simulink library "cfr_3fir_lib"  (Simulink 8.7)
settings: Solver=ode45  StartTime=0.0  StopTime=10.0  RelTol=1e-3
undefined symbols (not defined in the file): AdvDSPBChannelOutDisplay, Anti, cfr0_id, cfr_Params, clock_rate, dpoly, dspba_ChannelInVis, dspba_ChannelOutVis, dspba_internal_get_channel_ports, evalAionMaskParam, Folding, latency, primtype, REG, REG_dut_id_addr, sample_rate, Symmetrical, value
libraries: DSPBAPrim x83, CORDIC_lib x17, Pipereg_lib x15, DSPBAModelBus x3, DSPBAFilters x3
(part 1 of 2)
settings Model: Creator=nsafari  LastModifiedBy=5g

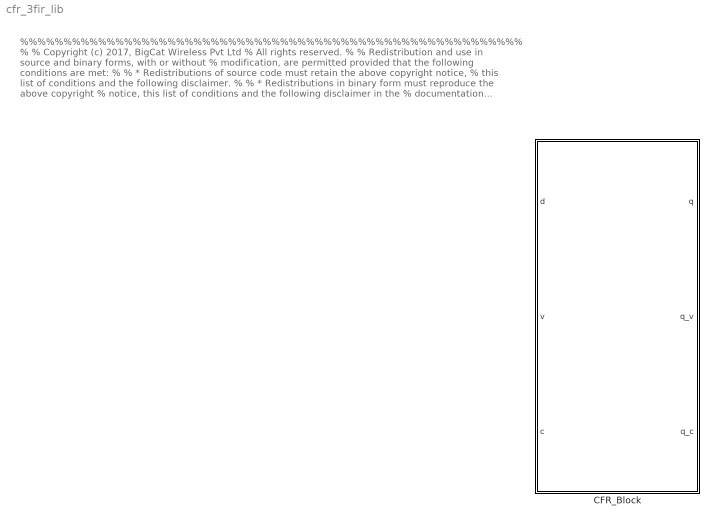
== system cfr_3fir_lib ==
  note: %%%%%%%%%%%%%%%%%%%%%%%%%%%%%%%%%%%%%%%%%%%%%%%%%%%%%%%%%%
      | %
      | % Copyright (c) 2017, BigCat Wireless Pvt Ltd
      | % All rights reserved.
      | %
      | % Redistribution and use in source and binary forms, with or without
      | % modification, are permitted provided that the following conditions are met:
      | %
      | % * Redistributions of source code must retain the above copyright notice,
      | % this list of conditions and the following disclaimer.
      | %
      | % * Redistributions in binary form must reproduce the above copyright
      | % notice, this list of conditions and the following disclaimer in the
      | % documentation and/or other materials provided with the distribution.
      | %
      | % * Neither the name of the copyright holder nor the names of its contributors
      | % may be used to endorse or promote products derived from this software
      | % without specific prior written permission.
      | %
      | %
      | %
      | % THIS SOFTWARE IS PROVIDED BY THE COPYRIGHT HOLDERS AND CONTRIBUTORS "AS IS"
      | % AND ANY EXPRESS OR IMPLIED WARRANTIES, INCLUDING, BUT NOT LIMITED TO, THE
      | % IMPLIED WARRANTIES OF MERCHANTABILITY AND FITNESS FOR A PARTICULAR PURPOSE ARE
      | % DISCLAIMED. IN NO EVENT SHALL THE COPYRIGHT HOLDER OR CONTRIBUTORS BE LIABLE
      | % FOR ANY DIRECT, INDIRECT, INCIDENTAL, SPECIAL, EXEMPLARY, OR CONSEQUENTIAL
      | % DAMAGES (INCLUDING, BUT NOT LIMITED TO, PROCUREMENT OF SUBSTITUTE GOODS OR
      | % SERVICES; LOSS OF USE, DATA, OR PROFITS; OR BUSINESS INTERRUPTION) HOWEVER
      | % CAUSED AND ON ANY THEORY OF LIABILITY, WHETHER IN CONTRACT, STRICT LIABILITY,
      | % OR TORT (INCLUDING NEGLIGENCE OR OTHERWISE) ARISING IN ANY WAY OUT OF THE USE
      | % OF THIS SOFTWARE, EVEN IF ADVISED OF THE POSSIBILITY OF SUCH DAMAGE.
      | %
      | %%%%%%%%%%%%%%%%%%%%%%%%%%%%%%%%%%%%%%%%%%%%%%%%%%%%%%%%%%
  CFR_Block : Subsystem  mask(Altera CFR Library Block){clk=clock_rate, sample_rate=sample_rate, Folding=Folding, block_id=cfr0_id, block_id_addr=REG_dut_id_addr, cfr_Params=cfr_Params(1), REG=REG, Pipeline_stages=0, ClockMargin=0, Pipeline_stages_actual_data=0}
      mask prompts: clk "System clock"; sample_rate "sample rate"; Folding "Folding Factor"; block_id "Unique ID of CFR"; block_id_addr "CFR ID address"; cfr_Params "CFR Configuration Structure"; REG "Register Map"
      mask help:
      | The block has the following parameters:
      |
      | "system clock" - the clock rate CFR module runs.
      |
      | "sample rate" - input signal sampling rate.
      |
      | "Folding Factor" - the number of folding for the module time-sharing;
      | It takes integer values between 1 and floor(system clock / sample rate).
      |
      | "Unique ID of CFR" is a unique numerical integer identifier for the CFR
      | block, this is used once the block is in a larger system to confirm the
      | correct block is being accessed.
      |
      | "CFR ID address" this is the relative address of the "Unique ID of CFR"
      | typically this is zero (at the CFR base address).
      |
      | "CFR Configuration Structure" - an array structure containing the
      | configuration of the CFR block. The length of this parameter specifies the
      | number of CFR core iterations instantiated.
      |
      | "Register Map" a structure containing the register map for CFR block.
      |
      | The settings of the above are exemplified in the setup script of the
      | altera_cfr example design.
      mask init:
      | %setup_cfr_block(iters, Iter_Params, REG, block_id, block_id_addr);
      mask Display:
      | fprintf('FIR-based \n Peak Cancelling CFR \n \n Folding Factor: %d\n', Folding);
      | port_label('input',1,'d');
      | port_label('input',2,'v');
      | port_label('input',3,'c');
      | port_label('output',1,'q');
      | port_label('output',2,'q_v');
      | port_label('output',3,'q_c');

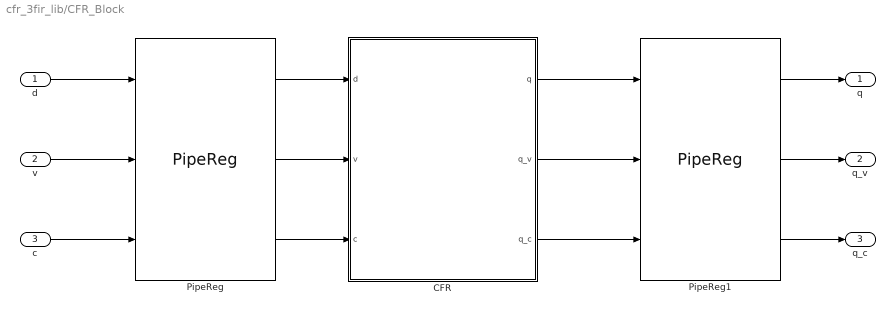
== system cfr_3fir_lib/CFR_Block ==
  d : Inport
  v : Inport  Port=2
  c : Inport  Port=3
  CFR : Subsystem
  PipeReg : Pipereg_lib/PipeReg  NPipe=Pipeline_stages  Clock_Margin=ClockMargin
  PipeReg1 : Pipereg_lib/PipeReg  NPipe=Pipeline_stages  Clock_Margin=ClockMargin
  q : Outport
  q_v : Outport  Port=2
  q_c : Outport  Port=3
  wires:
  v/1 -> PipeReg/2
  c/1 -> PipeReg/3
  d/1 -> PipeReg/1
  PipeReg1/2 -> q_v/1
  PipeReg1/3 -> q_c/1
  PipeReg1/1 -> q/1
  PipeReg/3 -> CFR/3(c)
  PipeReg/1 -> CFR/1(d)
  PipeReg/2 -> CFR/2(v)
  CFR/2(q_v) -> PipeReg1/2
  CFR/3(q_c) -> PipeReg1/3
  CFR/1(q) -> PipeReg1/1

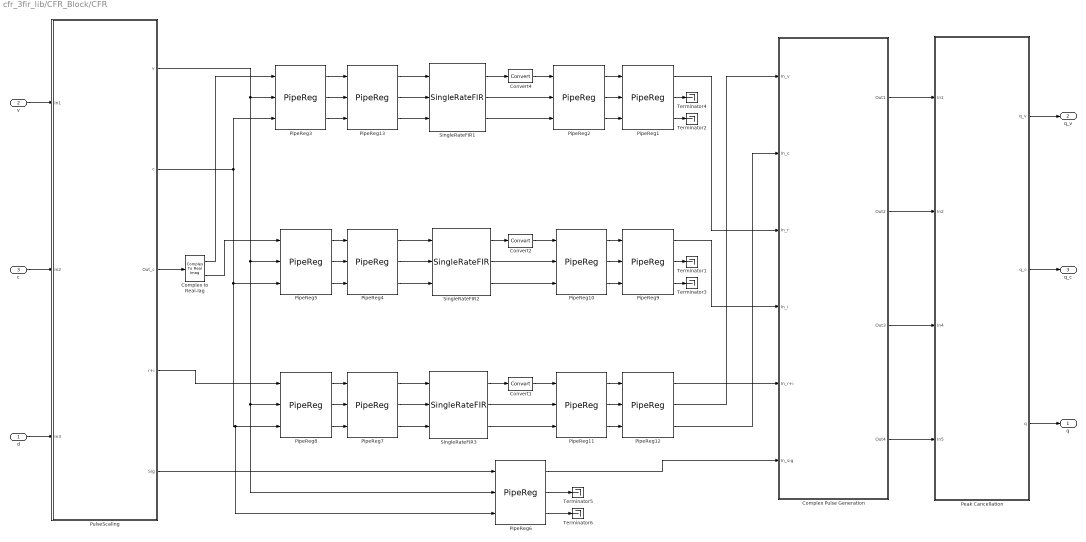
== system cfr_3fir_lib/CFR_Block/CFR ==
  d : Inport
  v : Inport  Port=2
  c : Inport  Port=3
  Complex Pulse Generation : Subsystem
  Complex to Real-Iag : ComplexToRealImag
  Convert1 : DSPBAPrim/Convert  primtype=convert  nInputs=1  nOutputs=1  omode=Specify via dialog  otype=sfix(16)  scale=2^-15  rndmethod=Unbiased  factor=1  satmethod=None  shift_vec=[0 1 2 -1]  value=round([0:255]/17)  inPortNames=[' '; ' ';]  outPortNames=[' '; 'c']  dspbaimage=dspba_prim.jpg  text=fprintf('convert');  style=Optimised  visibilities=8+64+256+2^17  clipdetect=off  floatPrecision=float32_m23  advOptions=[]  version=20130211
  Convert2 : DSPBAPrim/Convert  primtype=convert  nInputs=1  nOutputs=1  omode=Specify via dialog  otype=sfix(16)  scale=2^-15  rndmethod=Unbiased  factor=1  satmethod=None  shift_vec=[0 1 2 -1]  value=round([0:255]/17)  inPortNames=[' '; ' ';]  outPortNames=[' '; 'c']  dspbaimage=dspba_prim.jpg  text=fprintf('convert');  style=Optimised  visibilities=8+64+256+2^17  clipdetect=off  floatPrecision=float32_m23  advOptions=[]  version=20130211
  Convert4 : DSPBAPrim/Convert  primtype=convert  nInputs=1  nOutputs=1  omode=Specify via dialog  otype=sfix(16)  scale=2^-15  rndmethod=Unbiased  factor=1  satmethod=None  shift_vec=[0 1 2 -1]  value=round([0:255]/17)  inPortNames=[' '; ' ';]  outPortNames=[' '; 'c']  dspbaimage=dspba_prim.jpg  text=fprintf('convert');  style=Optimised  visibilities=8+64+256+2^17  clipdetect=off  floatPrecision=float32_m23  advOptions=[]  version=20130211
  Peak Cancellation : Subsystem
  PipeReg{1..5,7..13} (12 alike) : Pipereg_lib/PipeReg  NPipe=Pipeline_stages  Clock_Margin=ClockMargin
  PipeReg6 : Pipereg_lib/PipeReg  NPipe=Pipeline_stages_actual_data  Clock_Margin=ClockMargin
  PulseScaling : Subsystem
  SingleRateFIR1 : DSPBAFilters/SingleRateFIR  nInputRate=sample_rate  nchan=Folding  symmetry=Symmetrical  coef=fi(real(cfr_Params.firCOEF)/norm(cfr_Params.firCOEF),1,16,15)  addr=cfr_Params.BaseAddr + REG.FirTap1  rwmode=Read/Write  nband=Use All Taps  latency=4  exposebus=off  version=20090407
      settings: AttributesFormatString=%<latency>
  SingleRateFIR2 : DSPBAFilters/SingleRateFIR  nInputRate=sample_rate  nchan=Folding  symmetry=Anti-Symmetrical  coef=fi(imag(cfr_Params.firCOEF)/norm(cfr_Params.firCOEF),1,16,15)  addr=cfr_Params.BaseAddr + REG.FirTap2  rwmode=Constant  nband=Use All Taps  latency=4  exposebus=off  version=20090407
      settings: AttributesFormatString=%<latency>
  SingleRateFIR3 : DSPBAFilters/SingleRateFIR  nInputRate=sample_rate  nchan=Folding  symmetry=Non Symmetrical  coef=fi(real(cfr_Params.firCOEF)/norm(cfr_Params.firCOEF)+imag(cfr_Params.firCOEF)/norm(cfr_Params.firCOEF),1,16,15)  addr=cfr_Params.BaseAddr + REG.FirTap3  rwmode=Read/Write  nband=Use All Taps  latency=4  exposebus=off  version=20090407
      settings: AttributesFormatString=%<latency>
  Terminator{1..6} (6 alike) : Terminator
  q : Outport
  q_v : Outport  Port=2
  q_c : Outport  Port=3
  wires:
  Complex Pulse Generation/3(Out3) -> Peak Cancellation/3(In4)
  PipeReg1/3 -> Terminator2/1
  PipeReg12/2 -> Complex Pulse Generation/1(In_v)
  PipeReg9/1 -> Complex Pulse Generation/4(In_i)
  SingleRateFIR3/3 -> PipeReg11/3
  PipeReg2/3 -> PipeReg1/3
  SingleRateFIR2/1 -> Convert2/1
  PipeReg13/2 -> SingleRateFIR1/2
  PipeReg4/2 -> SingleRateFIR2/2
  Complex to Real-Iag/1 -> PipeReg3/1
  SingleRateFIR2/3 -> PipeReg10/3
  c/1 -> PulseScaling/2(In2)
  v/1 -> PulseScaling/1(In1)
  Complex Pulse Generation/4(Out4) -> Peak Cancellation/4(In5)
  SingleRateFIR3/1 -> Convert1/1
  PulseScaling/4(r+i) -> PipeReg8/1
  PulseScaling/1(v) -> PipeReg3/2, PipeReg5/2, PipeReg6/2, PipeReg8/2
  PipeReg11/2 -> PipeReg12/2
  PipeReg4/1 -> SingleRateFIR2/1
  Peak Cancellation/1(q_v) -> q_v/1
  Complex Pulse Generation/2(Out2) -> Peak Cancellation/2(In2)
  PipeReg2/1 -> PipeReg1/1
  PipeReg3/2 -> PipeReg13/2
  PipeReg12/3 -> Complex Pulse Generation/2(In_c)
  PipeReg8/2 -> PipeReg7/2
  PipeReg8/1 -> PipeReg7/1
  PipeReg13/1 -> SingleRateFIR1/1
  SingleRateFIR2/2 -> PipeReg10/2
  PipeReg6/3 -> Terminator6/1
  PipeReg7/2 -> SingleRateFIR3/2
  PulseScaling/3(Out_c) -> Complex to Real-Iag/1
  SingleRateFIR1/3 -> PipeReg2/3
  PipeReg9/2 -> Terminator1/1
  PipeReg2/2 -> PipeReg1/2
  PipeReg1/2 -> Terminator4/1
  d/1 -> PulseScaling/3(In3)
  PipeReg3/1 -> PipeReg13/1
  PulseScaling/2(c) -> PipeReg3/3, PipeReg5/3, PipeReg6/3, PipeReg8/3
  Complex Pulse Generation/1(Out1) -> Peak Cancellation/1(In1)
  PipeReg12/1 -> Complex Pulse Generation/5(In_r+i)
  PipeReg6/1 -> Complex Pulse Generation/6(In_sig)
  PipeReg7/3 -> SingleRateFIR3/3
  PipeReg3/3 -> PipeReg13/3
  Peak Cancellation/3(q) -> q/1
  PipeReg7/1 -> SingleRateFIR3/1
  Complex to Real-Iag/2 -> PipeReg5/1
  PipeReg4/3 -> SingleRateFIR2/3
  PipeReg6/2 -> Terminator5/1
  Convert2/1 -> PipeReg10/1
  PipeReg9/3 -> Terminator3/1
  Peak Cancellation/2(q_c) -> q_c/1
  PipeReg10/2 -> PipeReg9/2
  PipeReg8/3 -> PipeReg7/3
  PulseScaling/5(Sig) -> PipeReg6/1
  PipeReg11/1 -> PipeReg12/1
  SingleRateFIR1/1 -> Convert4/1
  PipeReg13/3 -> SingleRateFIR1/3
  PipeReg5/3 -> PipeReg4/3
  PipeReg5/2 -> PipeReg4/2
  PipeReg11/3 -> PipeReg12/3
  Convert4/1 -> PipeReg2/1
  PipeReg1/1 -> Complex Pulse Generation/3(In_r)
  Convert1/1 -> PipeReg11/1
  SingleRateFIR3/2 -> PipeReg11/2
  PipeReg5/1 -> PipeReg4/1
  SingleRateFIR1/2 -> PipeReg2/2
  PipeReg10/1 -> PipeReg9/1
  PipeReg10/3 -> PipeReg9/3

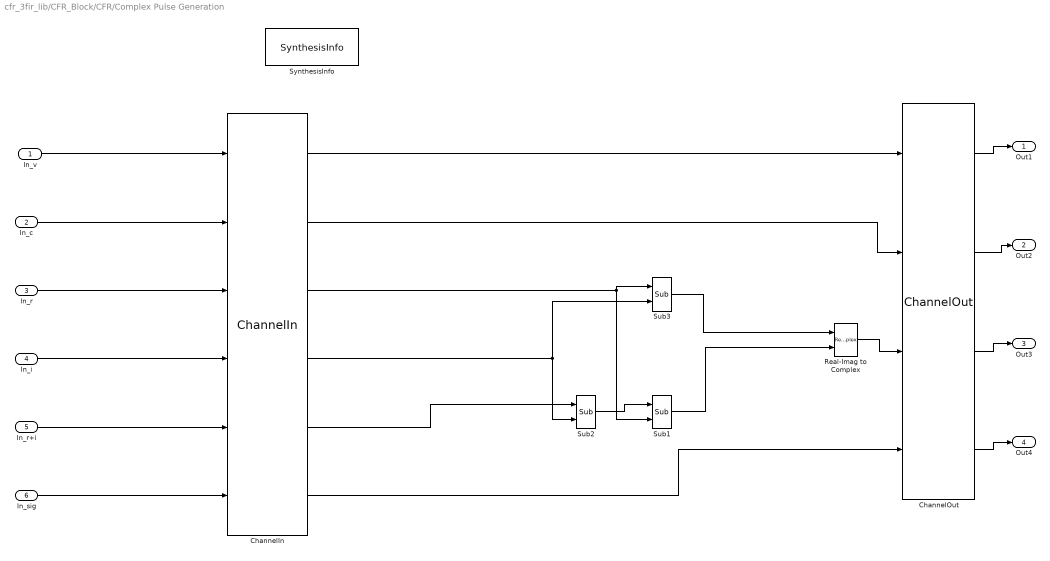
== system cfr_3fir_lib/CFR_Block/CFR/Complex Pulse Generation ==
  In_v : Inport
  In_c : Inport  Port=2
  In_r : Inport  Port=3
  In_i : Inport  Port=4
  In_r+i : Inport  Port=5
  In_sig : Inport  Port=6
  ChannelIn : DSPBAPrim/ChannelIn  primtype=channelin  nInputs=dspba_internal_get_channel_ports(gcb)  nOutputs=dspba_internal_get_channel_ports(gcb)  omode=Inherit via internal rule  otype=sfix(16)  scale=2^-15  rndmethod=Unbiased  factor=1  satmethod=Symmetric  shift_vec=[0 1 2 -1]  value=4  inPortNames=['v'; 'c'; '0'; '1'; '2'; '3'; '4'; '5'; '6'; '7'; '8'; '9'; 'A'; 'B'; 'D'; 'E'; 'F'; 'G'; 'H'; 'I'; 'J'; 'K'; 'L'; 'M'; 'N'; 'O'; 'P'; 'Q'; 'R'; 'S'; 'T'; 'U'; 'W'; 'X'; 'Y'; 'Z']  outPortNames=['v'; 'c'; '0'; '1'; '2'; '3'; '4'; '5'; '6'; '7'; '8'; '9'; 'A'; 'B'; 'D'; 'E'; 'F'; 'G'; 'H'; 'I'; 'J'; 'K'; 'L'; 'M'; 'N'; 'O'; 'P'; 'Q'; 'R'; 'S'; 'T'; 'U'; 'W'; 'X'; 'Y'; 'Z']  dspbaimage=dspba_prim.jpg  text=fprintf('In');  style=Optimised  dataSignals=4  foldingEnabled=off  channels=1  sampleRate=200  packetBeginPresent=off  packetBeginEnabled=off  visibilities=dspba_ChannelInVis(gcb)  latencyCorrection=0  version=20141013
  ChannelOut : DSPBAPrim/ChannelOut  primtype=channelout  nInputs=dspba_internal_get_channel_ports(gcb)  nOutputs=dspba_internal_get_channel_ports(gcb)  omode=Inherit via internal rule  otype=sfix(16)  scale=2^-15  rndmethod=Unbiased  factor=1  satmethod=Symmetric  shift_vec=[0 1 2 -1]  value=2  inPortNames=['v'; 'c'; '0'; '1'; '2'; '3'; '4'; '5'; '6'; '7'; '8'; '9'; 'A'; 'B'; 'D'; 'E'; 'F'; 'G'; 'H'; 'I'; 'J'; 'K'; 'L'; 'M'; 'N'; 'O'; 'P'; 'Q'; 'R'; 'S'; 'T'; 'U'; 'W'; 'X'; 'Y'; 'Z']  outPortNames=['v'; 'c'; '0'; '1'; '2'; '3'; '4'; '5'; '6'; '7'; '8'; '9'; 'A'; 'B'; 'D'; 'E'; 'F'; 'G'; 'H'; 'I'; 'J'; 'K'; 'L'; 'M'; 'N'; 'O'; 'P'; 'Q'; 'R'; 'S'; 'T'; 'U'; 'W'; 'X'; 'Y'; 'Z']  dspbaimage=dspba_prim.jpg  text=fprintf('Out%s', AdvDSPBChannelOutDisplay(latency));  style=Optimised  dataSignals=2  foldingEnabled=off  channels=1  sampleRate=200  packetBeginPresent=off  packetBeginEnabled=off  visibilities=dspba_ChannelOutVis(gcb)  latency=2  latencyCorrection=0  version=20141013
  Real-Imag to Complex : RealImagToComplex
  Sub1 : DSPBAPrim/Sub  primtype=sub  nInputs=2  nOutputs=1  omode=Specify via dialog  otype=sfix(16)  scale=2^-15  rndmethod=Unbiased  factor=1  satmethod=Symmetric  shift_vec=[0 1 2 -1]  value=0  inPortNames=['+'; '-';]  outPortNames=[' ']  dspbaimage=dspba_prim.jpg  text=fprintf('-');  style=Optimised  visibilities=8  floatRounding=correct  advOptions=[]  version=20130115
  Sub2 : DSPBAPrim/Sub  primtype=sub  nInputs=2  nOutputs=1  omode=Specify via dialog  otype=sfix(16)  scale=2^-15  rndmethod=Unbiased  factor=1  satmethod=Symmetric  shift_vec=[0 1 2 -1]  value=0  inPortNames=['+'; '-';]  outPortNames=[' ']  dspbaimage=dspba_prim.jpg  text=fprintf('-');  style=Optimised  visibilities=8  floatRounding=correct  advOptions=[]  version=20130115
  Sub3 : DSPBAPrim/Sub  primtype=sub  nInputs=2  nOutputs=1  omode=Specify via dialog  otype=sfix(16)  scale=2^-15  rndmethod=Unbiased  factor=1  satmethod=Symmetric  shift_vec=[0 1 2 -1]  value=0  inPortNames=['+'; '-';]  outPortNames=[' ']  dspbaimage=dspba_prim.jpg  text=fprintf('-');  style=Optimised  visibilities=8  floatRounding=correct  advOptions=[]  version=20130115
  SynthesisInfo : DSPBAPrim/SynthesisInfo  primtype=synthinfo  nInputs=0  nOutputs=0  omode=Inherit via internal rule  otype=sfix(16)  scale=2^-15  rndmethod=Truncate  factor=1  satmethod=Symmetric  shift_vec=[0 1 2 -1]  value=99  inPortNames=[' '; ' ';]  outPortNames=[' ']  dspbaimage=dspba_prim.jpg  text=fprintf('Style=%s', style);  style=Scheduled  visibilities=32768  constraintInUse=on  constraintRelation=>  constraintLimit=5  bitAccurate=off  version=20090407
  Out1 : Outport
  Out2 : Outport  Port=2
  Out3 : Outport  Port=3
  Out4 : Outport  Port=4
  wires:
  Sub2/1 -> Sub1/1
  ChannelOut/2 -> Out2/1
  ChannelIn/3 -> Sub1/2, Sub3/1
  ChannelIn/4 -> Sub2/2, Sub3/2
  ChannelIn/5 -> Sub2/1
  Sub1/1 -> Real-Imag to Complex/2
  Real-Imag to Complex/1 -> ChannelOut/3
  ChannelOut/3 -> Out3/1
  ChannelOut/4 -> Out4/1
  ChannelOut/1 -> Out1/1
  Sub3/1 -> Real-Imag to Complex/1
  ChannelIn/6 -> ChannelOut/4
  In_v/1 -> ChannelIn/1
  In_r+i/1 -> ChannelIn/5
  In_sig/1 -> ChannelIn/6
  ChannelIn/2 -> ChannelOut/2
  ChannelIn/1 -> ChannelOut/1
  In_c/1 -> ChannelIn/2
  In_i/1 -> ChannelIn/4
  In_r/1 -> ChannelIn/3

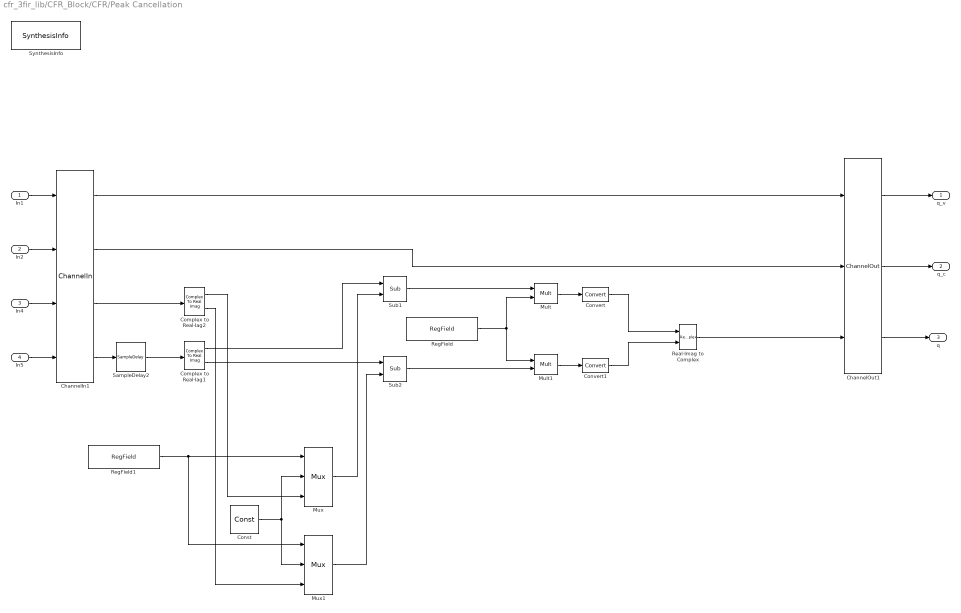
== system cfr_3fir_lib/CFR_Block/CFR/Peak Cancellation ==
  In1 : Inport
  In2 : Inport  Port=2
  In4 : Inport  Port=3
  In5 : Inport  Port=4
  ChannelIn1 : DSPBAPrim/ChannelIn  primtype=channelin  nInputs=dspba_internal_get_channel_ports(gcb)  nOutputs=dspba_internal_get_channel_ports(gcb)  omode=Inherit via internal rule  otype=sfix(16)  scale=2^-15  rndmethod=Unbiased  factor=1  satmethod=Symmetric  shift_vec=[0 1 2 -1]  value=2  inPortNames=['v'; 'c'; '0'; '1'; '2'; '3'; '4'; '5'; '6'; '7'; '8'; '9'; 'A'; 'B'; 'D'; 'E'; 'F'; 'G'; 'H'; 'I'; 'J'; 'K'; 'L'; 'M'; 'N'; 'O'; 'P'; 'Q'; 'R'; 'S'; 'T'; 'U'; 'W'; 'X'; 'Y'; 'Z']  outPortNames=['v'; 'c'; '0'; '1'; '2'; '3'; '4'; '5'; '6'; '7'; '8'; '9'; 'A'; 'B'; 'D'; 'E'; 'F'; 'G'; 'H'; 'I'; 'J'; 'K'; 'L'; 'M'; 'N'; 'O'; 'P'; 'Q'; 'R'; 'S'; 'T'; 'U'; 'W'; 'X'; 'Y'; 'Z']  dspbaimage=dspba_prim.jpg  text=fprintf('In');  style=Optimised  dataSignals=2  foldingEnabled=off  channels=1  sampleRate=200  packetBeginPresent=off  packetBeginEnabled=off  visibilities=dspba_ChannelInVis(gcb)  latencyCorrection=0  version=20141013
  ChannelOut1 : DSPBAPrim/ChannelOut  primtype=channelout  nInputs=dspba_internal_get_channel_ports(gcb)  nOutputs=dspba_internal_get_channel_ports(gcb)  omode=Inherit via internal rule  otype=sfix(16)  scale=2^-15  rndmethod=Unbiased  factor=1  satmethod=Symmetric  shift_vec=[0 1 2 -1]  value=1  inPortNames=['v'; 'c'; '0'; '1'; '2'; '3'; '4'; '5'; '6'; '7'; '8'; '9'; 'A'; 'B'; 'D'; 'E'; 'F'; 'G'; 'H'; 'I'; 'J'; 'K'; 'L'; 'M'; 'N'; 'O'; 'P'; 'Q'; 'R'; 'S'; 'T'; 'U'; 'W'; 'X'; 'Y'; 'Z']  outPortNames=['v'; 'c'; '0'; '1'; '2'; '3'; '4'; '5'; '6'; '7'; '8'; '9'; 'A'; 'B'; 'D'; 'E'; 'F'; 'G'; 'H'; 'I'; 'J'; 'K'; 'L'; 'M'; 'N'; 'O'; 'P'; 'Q'; 'R'; 'S'; 'T'; 'U'; 'W'; 'X'; 'Y'; 'Z']  dspbaimage=dspba_prim.jpg  text=fprintf('Out%s', AdvDSPBChannelOutDisplay(latency));  style=Optimised  dataSignals=1  foldingEnabled=off  channels=1  sampleRate=200  packetBeginPresent=off  packetBeginEnabled=off  visibilities=dspba_ChannelOutVis(gcb)  latency=8  latencyCorrection=0  version=20141013
  Complex to Real-Iag1 : ComplexToRealImag
  Complex to Real-Iag2 : ComplexToRealImag
  Const : DSPBAPrim/Const  primtype=const  nInputs=0  nOutputs=1  omode=Inherit via internal rule  otype=sfix(16)  scale=2^-15  rndmethod=Unbiased  factor=1  satmethod=Symmetric  shift_vec=[0 1 2 -1]  value=0  inPortNames=['+'; '+';]  outPortNames=[' ']  dspbaimage=dspba_prim.jpg  text=fprintf('%s', num2str(value));  style=Optimised  visibilities=8 + 1024  floatPrecision=float32_m23  version=20120820
  Convert : DSPBAPrim/Convert  primtype=convert  nInputs=1  nOutputs=1  omode=Specify via dialog  otype=sfix(16)  scale=2^-15  rndmethod=Unbiased  factor=1  satmethod=None  shift_vec=[0 1 2 -1]  value=round([0:255]/17)  inPortNames=[' '; ' ';]  outPortNames=[' '; 'c']  dspbaimage=dspba_prim.jpg  text=fprintf('convert');  style=Optimised  visibilities=8+64+256+2^17  clipdetect=off  floatPrecision=float32_m23  advOptions=[]  version=20130211
  Convert1 : DSPBAPrim/Convert  primtype=convert  nInputs=1  nOutputs=1  omode=Specify via dialog  otype=sfix(16)  scale=2^-15  rndmethod=Unbiased  factor=1  satmethod=None  shift_vec=[0 1 2 -1]  value=round([0:255]/17)  inPortNames=[' '; ' ';]  outPortNames=[' '; 'c']  dspbaimage=dspba_prim.jpg  text=fprintf('convert');  style=Optimised  visibilities=8+64+256+2^17  clipdetect=off  floatPrecision=float32_m23  advOptions=[]  version=20130211
  Mult : DSPBAPrim/Mult  primtype=mult  nInputs=2  nOutputs=1  omode=Inherit via internal rule  otype=sfix(16)  scale=2^-15  rndmethod=Unbiased  factor=1  satmethod=Symmetric  shift_vec=[0 1 2 -1]  value=0  inPortNames=[' '; ' ';]  outPortNames=[' ']  dspbaimage=dspba_prim.jpg  text=fprintf('X');  style=Optimised  visibilities=8+2^18+2^19  floatPrecision=float32_m23  floatRounding=correct  advOptions=[]  version=20130115
  Mult1 : DSPBAPrim/Mult  primtype=mult  nInputs=2  nOutputs=1  omode=Inherit via internal rule  otype=sfix(16)  scale=2^-15  rndmethod=Unbiased  factor=1  satmethod=Symmetric  shift_vec=[0 1 2 -1]  value=0  inPortNames=[' '; ' ';]  outPortNames=[' ']  dspbaimage=dspba_prim.jpg  text=fprintf('X');  style=Optimised  visibilities=8+2^18+2^19  floatPrecision=float32_m23  floatRounding=correct  advOptions=[]  version=20130115
  Mux : DSPBAPrim/Mux  primtype=mux  nInputs=evalAionMaskParam(gcb,'value',1)+1  nOutputs=1  omode=Inherit via internal rule  otype=sfix(16)  scale=2^-15  rndmethod=Unbiased  factor=1  satmethod=Symmetric  shift_vec=[0 1 2 -1]  value=2  inPortNames=['s '; 'd0'; 'd1'; 'd2'; 'd3'; 'd4'; 'd5'; 'd6'; 'd7'; 'd8'; 'd9';]  outPortNames=[' ']  dspbaimage=dspba_prim.jpg  text=fprintf('%s', primtype);  style=Optimised  visibilities=1032  version=20131025
  Mux1 : DSPBAPrim/Mux  primtype=mux  nInputs=evalAionMaskParam(gcb,'value',1)+1  nOutputs=1  omode=Inherit via internal rule  otype=sfix(16)  scale=2^-15  rndmethod=Unbiased  factor=1  satmethod=Symmetric  shift_vec=[0 1 2 -1]  value=2  inPortNames=['s '; 'd0'; 'd1'; 'd2'; 'd3'; 'd4'; 'd5'; 'd6'; 'd7'; 'd8'; 'd9';]  outPortNames=[' ']  dspbaimage=dspba_prim.jpg  text=fprintf('%s', primtype);  style=Optimised  visibilities=1032  version=20131025
  Real-Imag to Complex : RealImagToComplex
  RegField : DSPBAModelBus/RegField  reg_name=cfr_Params.BaseAddr + REG.Scaling  reg_rwmode=Read/Write  reg_msb=15  reg_lsb=0  reg_mode=Specify via dialog  reg_type=ufix(9)  reg_scale=2^-8  reg_init=cfr_Params.Scaling  reg_desc=Scaling value  reg_modal=off  reg_desc0=0  reg_desc1=0  reg_desc2=0  reg_desc3=0  reg_desc4=0  reg_desc5=0  reg_desc6=0  reg_desc7=0  SampleTime=1  version=20090407
  RegField1 : DSPBAModelBus/RegField  reg_name=cfr_Params.BaseAddr + REG.Enable  reg_rwmode=Read/Write  reg_msb=0  reg_lsb=0  reg_mode=Specify via dialog  reg_type=ufix(1)  reg_scale=2^0  reg_init=cfr_Params.Enable  reg_desc=Enable CFR  reg_modal=off  reg_desc0=0  reg_desc1=0  reg_desc2=0  reg_desc3=0  reg_desc4=0  reg_desc5=0  reg_desc6=0  reg_desc7=0  SampleTime=1  version=20090407
  SampleDelay2 : DSPBAPrim/SampleDelay  primtype=sampdelay  nInputs=1  nOutputs=1  omode=Inherit via internal rule  otype=sfix(16)  scale=2^-15  rndmethod=Unbiased  factor=1  satmethod=Symmetric  shift_vec=[0 1 2 -1]  value=(floor(length(cfr_Params.firCOEF)/2)*Folding)  inPortNames=[' '; ' ';]  outPortNames=[' ']  dspbaimage=dspba_prim.jpg  text=dpoly(1, eye(1,value+1), 'z')  style=Optimised  visibilities=8 + 1024 + 2^17 + 2^18  flexible=off  slackgroup=0  augmented=0  version=20090407  advOptions=[]
  Sub1 : DSPBAPrim/Sub  primtype=sub  nInputs=2  nOutputs=1  omode=Inherit via internal rule  otype=sfix(16)  scale=2^-15  rndmethod=Unbiased  factor=1  satmethod=Symmetric  shift_vec=[0 1 2 -1]  value=0  inPortNames=['+'; '-';]  outPortNames=[' ']  dspbaimage=dspba_prim.jpg  text=fprintf('-');  style=Optimised  visibilities=8  floatRounding=correct  advOptions=[]  version=20130115
  Sub2 : DSPBAPrim/Sub  primtype=sub  nInputs=2  nOutputs=1  omode=Inherit via internal rule  otype=sfix(16)  scale=2^-15  rndmethod=Unbiased  factor=1  satmethod=Symmetric  shift_vec=[0 1 2 -1]  value=0  inPortNames=['+'; '-';]  outPortNames=[' ']  dspbaimage=dspba_prim.jpg  text=fprintf('-');  style=Optimised  visibilities=8  floatRounding=correct  advOptions=[]  version=20130115
  SynthesisInfo : DSPBAPrim/SynthesisInfo  primtype=synthinfo  nInputs=0  nOutputs=0  omode=Inherit via internal rule  otype=sfix(16)  scale=2^-15  rndmethod=Truncate  factor=1  satmethod=Symmetric  shift_vec=[0 1 2 -1]  value=99  inPortNames=[' '; ' ';]  outPortNames=[' ']  dspbaimage=dspba_prim.jpg  text=fprintf('Style=%s', style);  style=Scheduled  visibilities=32768  constraintInUse=on  constraintRelation=>  constraintLimit=12  bitAccurate=off  version=20090407
  q_v : Outport
  q_c : Outport  Port=2
  q : Outport  Port=3
  wires:
  Convert1/1 -> Real-Imag to Complex/2
  Convert/1 -> Real-Imag to Complex/1
  Sub2/1 -> Mult1/2
  Sub1/1 -> Mult/1
  Mult1/1 -> Convert1/1
  Mult/1 -> Convert/1
  RegField/1 -> Mult/2, Mult1/1
  SampleDelay2/1 -> Complex to Real-Iag1/1
  ChannelOut1/3 -> q/1
  ChannelOut1/2 -> q_c/1
  ChannelOut1/1 -> q_v/1
  In5/1 -> ChannelIn1/4
  In2/1 -> ChannelIn1/2
  In4/1 -> ChannelIn1/3
  In1/1 -> ChannelIn1/1
  ChannelIn1/2 -> ChannelOut1/2
  ChannelIn1/1 -> ChannelOut1/1
  Complex to Real-Iag1/2 -> Sub2/1
  Complex to Real-Iag1/1 -> Sub1/1
  Real-Imag to Complex/1 -> ChannelOut1/3
  ChannelIn1/4 -> SampleDelay2/1
  ChannelIn1/3 -> Complex to Real-Iag2/1
  RegField1/1 -> Mux/1, Mux1/1
  Complex to Real-Iag2/1 -> Mux/3
  Complex to Real-Iag2/2 -> Mux1/3
  Mux/1 -> Sub1/2
  Mux1/1 -> Sub2/2
  Const/1 -> Mux1/2, Mux/2

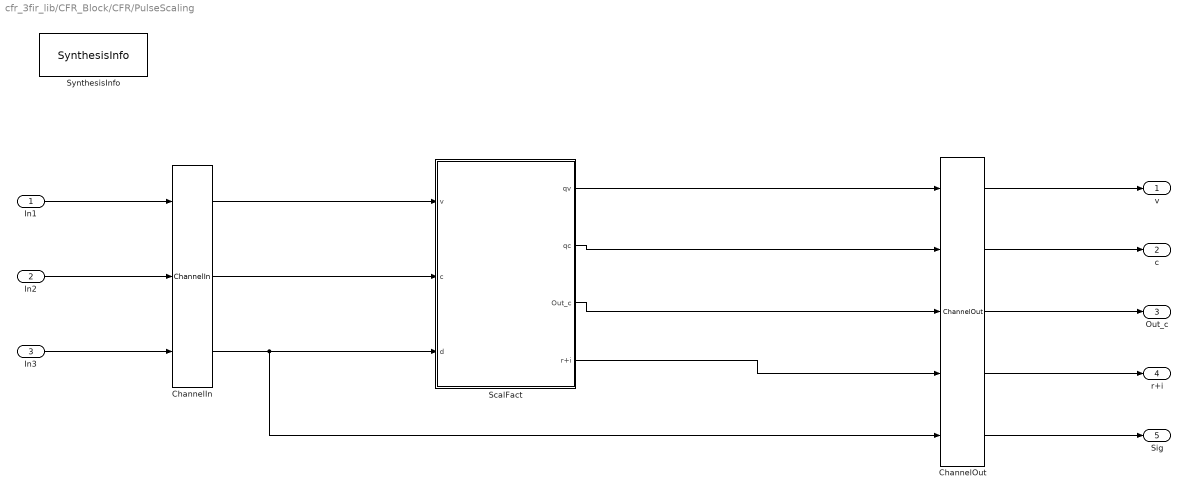
== system cfr_3fir_lib/CFR_Block/CFR/PulseScaling ==
  In1 : Inport
  In2 : Inport  Port=2
  In3 : Inport  Port=3
  ChannelIn : DSPBAPrim/ChannelIn  primtype=channelin  nInputs=dspba_internal_get_channel_ports(gcb)  nOutputs=dspba_internal_get_channel_ports(gcb)  omode=Inherit via internal rule  otype=sfix(16)  scale=2^-15  rndmethod=Unbiased  factor=1  satmethod=Symmetric  shift_vec=[0 1 2 -1]  value=1  inPortNames=['v'; 'c'; '0'; '1'; '2'; '3'; '4'; '5'; '6'; '7'; '8'; '9'; 'A'; 'B'; 'D'; 'E'; 'F'; 'G'; 'H'; 'I'; 'J'; 'K'; 'L'; 'M'; 'N'; 'O'; 'P'; 'Q'; 'R'; 'S'; 'T'; 'U'; 'W'; 'X'; 'Y'; 'Z']  outPortNames=['v'; 'c'; '0'; '1'; '2'; '3'; '4'; '5'; '6'; '7'; '8'; '9'; 'A'; 'B'; 'D'; 'E'; 'F'; 'G'; 'H'; 'I'; 'J'; 'K'; 'L'; 'M'; 'N'; 'O'; 'P'; 'Q'; 'R'; 'S'; 'T'; 'U'; 'W'; 'X'; 'Y'; 'Z']  dspbaimage=dspba_prim.jpg  text=fprintf('In');  style=Optimised  dataSignals=1  foldingEnabled=off  channels=1  sampleRate=200  packetBeginPresent=off  packetBeginEnabled=off  visibilities=dspba_ChannelInVis(gcb)  latencyCorrection=0  version=20141013
  ChannelOut : DSPBAPrim/ChannelOut  primtype=channelout  nInputs=dspba_internal_get_channel_ports(gcb)  nOutputs=dspba_internal_get_channel_ports(gcb)  omode=Inherit via internal rule  otype=sfix(16)  scale=2^-15  rndmethod=Unbiased  factor=1  satmethod=Symmetric  shift_vec=[0 1 2 -1]  value=3  inPortNames=['v'; 'c'; '0'; '1'; '2'; '3'; '4'; '5'; '6'; '7'; '8'; '9'; 'A'; 'B'; 'D'; 'E'; 'F'; 'G'; 'H'; 'I'; 'J'; 'K'; 'L'; 'M'; 'N'; 'O'; 'P'; 'Q'; 'R'; 'S'; 'T'; 'U'; 'W'; 'X'; 'Y'; 'Z']  outPortNames=['v'; 'c'; '0'; '1'; '2'; '3'; '4'; '5'; '6'; '7'; '8'; '9'; 'A'; 'B'; 'D'; 'E'; 'F'; 'G'; 'H'; 'I'; 'J'; 'K'; 'L'; 'M'; 'N'; 'O'; 'P'; 'Q'; 'R'; 'S'; 'T'; 'U'; 'W'; 'X'; 'Y'; 'Z']  dspbaimage=dspba_prim.jpg  text=fprintf('Out%s', AdvDSPBChannelOutDisplay(latency));  style=Optimised  dataSignals=3  foldingEnabled=off  channels=1  sampleRate=200  packetBeginPresent=off  packetBeginEnabled=off  visibilities=dspba_ChannelOutVis(gcb)  latency=40  latencyCorrection=0  version=20141013
  ScalFact : Subsystem  mask{ClipVal=cfr_Params.ClipVal}
      mask prompts: ClipVal "cLipping Value"
  SynthesisInfo : DSPBAPrim/SynthesisInfo  primtype=synthinfo  nInputs=0  nOutputs=0  omode=Inherit via internal rule  otype=sfix(16)  scale=2^-15  rndmethod=Truncate  factor=1  satmethod=Symmetric  shift_vec=[0 1 2 -1]  value=99  inPortNames=[' '; ' ';]  outPortNames=[' ']  dspbaimage=dspba_prim.jpg  text=fprintf('Style=%s', style);  style=Scheduled  visibilities=32768  constraintInUse=on  constraintRelation=>  constraintLimit=60  bitAccurate=off  version=20090407
  v : Outport
  c : Outport  Port=2
  Out_c : Outport  Port=3
  r+i : Outport  Port=4
  Sig : Outport  Port=5
  wires:
  ChannelOut/5 -> Sig/1
  ScalFact/4(r+i) -> ChannelOut/4
  ChannelOut/4 -> r+i/1
  ChannelOut/3 -> Out_c/1
  ChannelOut/2 -> c/1
  ChannelOut/1 -> v/1
  ChannelIn/3 -> ScalFact/3(d), ChannelOut/5
  ChannelIn/2 -> ScalFact/2(c)
  ChannelIn/1 -> ScalFact/1(v)
  In3/1 -> ChannelIn/3
  ScalFact/3(Out_c) -> ChannelOut/3
  ScalFact/2(qc) -> ChannelOut/2
  ScalFact/1(qv) -> ChannelOut/1
  In2/1 -> ChannelIn/2
  In1/1 -> ChannelIn/1

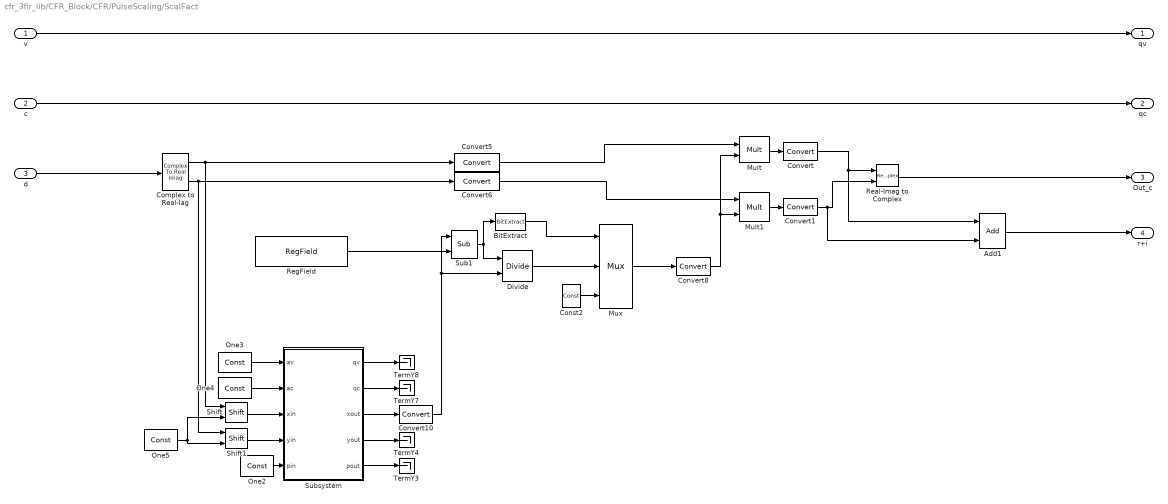
== system cfr_3fir_lib/CFR_Block/CFR/PulseScaling/ScalFact ==
  v : Inport
  c : Inport  Port=2
  d : Inport  Port=3
  Add1 : DSPBAPrim/Add  primtype=add  nInputs=evalAionMaskParam(gcb,'value',1)  nOutputs=1  omode=Inherit via internal rule with word growth  otype=sfix(16)  scale=2^-15  rndmethod=Unbiased  factor=1  satmethod=Symmetric  shift_vec=[0 1 2 -1]  value=2  inPortNames=[' '; ' ';]  outPortNames=[' ']  dspbaimage=dspba_prim.jpg  text=fprintf('+');  style=Optimised  visibilities=1032+2^17+2^18+2^19  genFPC=off  floatRounding=correct  advOptions=[]  version=20130821
  BitExtract : DSPBAPrim/BitExtract  primtype=bitextract  nInputs=1  nOutputs=1  omode=boolean  otype=sfix(16)  scale=1  rndmethod=Unbiased  factor=1  satmethod=Symmetric  shift_vec=[0 1 2 -1]  value=7  inPortNames=[' '; ' ';]  outPortNames=[' ']  dspbaimage=dspba_prim.jpg  text=fprintf('..%d', value);  style=Optimised  visibilities=8 + 1024  version=20090407
  Complex to Real-Iag : ComplexToRealImag
  Const2 : DSPBAPrim/Const  primtype=const  nInputs=0  nOutputs=1  omode=Inherit via internal rule  otype=sfix(16)  scale=2^-15  rndmethod=Unbiased  factor=1  satmethod=Symmetric  shift_vec=[0 1 2 -1]  value=0  inPortNames=['+'; '+';]  outPortNames=[' ']  dspbaimage=dspba_prim.jpg  text=fprintf('%s', num2str(value));  style=Optimised  visibilities=8 + 1024  floatPrecision=float32_m23  version=20120820
  Convert : DSPBAPrim/Convert  primtype=convert  nInputs=1  nOutputs=1  omode=Specify via dialog  otype=sfix(12)  scale=2^-11  rndmethod=Unbiased  factor=1  satmethod=None  shift_vec=[0 1 2 -1]  value=round([0:255]/17)  inPortNames=[' '; ' ';]  outPortNames=[' '; 'c']  dspbaimage=dspba_prim.jpg  text=fprintf('convert');  style=Optimised  visibilities=8+64+256+2^17  clipdetect=off  floatPrecision=float32_m23  advOptions=[]  version=20130211
  Convert1 : DSPBAPrim/Convert  primtype=convert  nInputs=1  nOutputs=1  omode=Specify via dialog  otype=sfix(12)  scale=2^-11  rndmethod=Unbiased  factor=1  satmethod=None  shift_vec=[0 1 2 -1]  value=round([0:255]/17)  inPortNames=[' '; ' ';]  outPortNames=[' '; 'c']  dspbaimage=dspba_prim.jpg  text=fprintf('convert');  style=Optimised  visibilities=8+64+256+2^17  clipdetect=off  floatPrecision=float32_m23  advOptions=[]  version=20130211
  Convert10 : DSPBAPrim/Convert  primtype=convert  nInputs=1  nOutputs=1  omode=Specify via dialog  otype=ufix(8)  scale=2^-6  rndmethod=Truncate  factor=1  satmethod=None  shift_vec=[0 1 2 -1]  value=round([0:255]/17)  inPortNames=[' '; ' ';]  outPortNames=[' '; 'c']  dspbaimage=dspba_prim.jpg  text=fprintf('convert');  style=Optimised  visibilities=8+64+256+2^17  clipdetect=off  floatPrecision=float32_m23  advOptions=[]  version=20130211
  Convert5 : DSPBAPrim/Convert  primtype=convert  nInputs=1  nOutputs=1  omode=Specify via dialog  otype=sfix(16)  scale=2^-15  rndmethod=Unbiased  factor=1  satmethod=None  shift_vec=[0 1 2 -1]  value=round([0:255]/17)  inPortNames=[' '; ' ';]  outPortNames=[' '; 'c']  dspbaimage=dspba_prim.jpg  text=fprintf('convert');  style=Optimised  visibilities=8+64+256+2^17  clipdetect=off  floatPrecision=float32_m23  advOptions=[]  version=20130211
  Convert6 : DSPBAPrim/Convert  primtype=convert  nInputs=1  nOutputs=1  omode=Specify via dialog  otype=sfix(16)  scale=2^-15  rndmethod=Unbiased  factor=1  satmethod=None  shift_vec=[0 1 2 -1]  value=round([0:255]/17)  inPortNames=[' '; ' ';]  outPortNames=[' '; 'c']  dspbaimage=dspba_prim.jpg  text=fprintf('convert');  style=Optimised  visibilities=8+64+256+2^17  clipdetect=off  floatPrecision=float32_m23  advOptions=[]  version=20130211
  Convert8 : DSPBAPrim/Convert  primtype=convert  nInputs=1  nOutputs=1  omode=Specify via dialog  otype=ufix(16)  scale=2^-15  rndmethod=Unbiased  factor=1  satmethod=None  shift_vec=[0 1 2 -1]  value=round([0:255]/17)  inPortNames=[' '; ' ';]  outPortNames=[' '; 'c']  dspbaimage=dspba_prim.jpg  text=fprintf('convert');  style=Optimised  visibilities=8+64+256+2^17  clipdetect=off  floatPrecision=float32_m23  advOptions=[]  version=20130211
  Divide : DSPBAPrim/Divide  primtype=divide  nInputs=2  nOutputs=1  omode=Inherit via internal rule  otype=ufix(16)  scale=2^-15  rndmethod=Unbiased  factor=1  satmethod=Symmetric  shift_vec=[0 1 2 -1]  value=round([0:255]/17)  inPortNames=[' '; ' ';]  outPortNames=[' ']  dspbaimage=dspba_prim.jpg  text=fprintf('a\n----\nb');  style=Optimised  visibilities=8+2^17+2^18  floatRounding=correct  advOptions=[]  version=20130115
  Mult : DSPBAPrim/Mult  primtype=mult  nInputs=2  nOutputs=1  omode=Inherit via internal rule  otype=sfix(16)  scale=2^-15  rndmethod=Unbiased  factor=1  satmethod=Symmetric  shift_vec=[0 1 2 -1]  value=0  inPortNames=[' '; ' ';]  outPortNames=[' ']  dspbaimage=dspba_prim.jpg  text=fprintf('X');  style=Optimised  visibilities=8+2^18+2^19  floatPrecision=float32_m23  floatRounding=correct  advOptions=[]  version=20130115
  Mult1 : DSPBAPrim/Mult  primtype=mult  nInputs=2  nOutputs=1  omode=Inherit via internal rule  otype=sfix(16)  scale=2^-15  rndmethod=Unbiased  factor=1  satmethod=Symmetric  shift_vec=[0 1 2 -1]  value=0  inPortNames=[' '; ' ';]  outPortNames=[' ']  dspbaimage=dspba_prim.jpg  text=fprintf('X');  style=Optimised  visibilities=8+2^18+2^19  floatPrecision=float32_m23  floatRounding=correct  advOptions=[]  version=20130115
  Mux : DSPBAPrim/Mux  primtype=mux  nInputs=evalAionMaskParam(gcb,'value',1)+1  nOutputs=1  omode=Inherit via internal rule  otype=sfix(16)  scale=2^-15  rndmethod=Unbiased  factor=1  satmethod=Symmetric  shift_vec=[0 1 2 -1]  value=2  inPortNames=['s'; 'd0'; 'd1'; 'd2'; 'd3'; 'd4'; 'd5'; 'd6'; 'd7'; 'd8'; 'd9';]  outPortNames=[' ']  dspbaimage=dspba_prim.jpg  text=fprintf('%s', primtype);  style=Optimised  visibilities=1032  version=20131025
  One2 : DSPBAPrim/Const  primtype=const  nInputs=0  nOutputs=1  omode=Specify via dialog  otype=sfix(18)  scale=2^-14  rndmethod=Unbiased  factor=1  satmethod=Symmetric  shift_vec=[0 1 2 -1]  value=0  inPortNames=['+'; '+';]  outPortNames=[' ']  dspbaimage=dspba_prim.jpg  text=fprintf('%s', num2str(value));  style=Optimised  visibilities=8 + 1024  floatPrecision=float32_m23  version=20120820
  One3 : DSPBAPrim/Const  primtype=const  nInputs=0  nOutputs=1  omode=boolean  otype=sfix(16)  scale=2^-15  rndmethod=Unbiased  factor=1  satmethod=Symmetric  shift_vec=[0 1 2 -1]  value=1  inPortNames=['+'; '+';]  outPortNames=[' ']  dspbaimage=dspba_prim.jpg  text=fprintf('%s', num2str(value));  style=Optimised  visibilities=8 + 1024  floatPrecision=float32_m23  version=20120820
  One4 : DSPBAPrim/Const  primtype=const  nInputs=0  nOutputs=1  omode=Specify via dialog  otype=uint(8)  scale=1  rndmethod=Unbiased  factor=1  satmethod=Symmetric  shift_vec=[0 1 2 -1]  value=0  inPortNames=['+'; '+';]  outPortNames=[' ']  dspbaimage=dspba_prim.jpg  text=fprintf('%s', num2str(value));  style=Optimised  visibilities=8 + 1024  floatPrecision=float32_m23  version=20120820
  One5 : DSPBAPrim/Const  primtype=const  nInputs=0  nOutputs=1  omode=Specify via dialog  otype=uint(4)  scale=2^0  rndmethod=Unbiased  factor=1  satmethod=Symmetric  shift_vec=[0 1 2 -1]  value=2  inPortNames=['+'; '+';]  outPortNames=[' ']  dspbaimage=dspba_prim.jpg  text=fprintf('%s', num2str(value));  style=Optimised  visibilities=8 + 1024  floatPrecision=float32_m23  version=20120820
  Real-Imag to Complex : RealImagToComplex
  RegField : DSPBAModelBus/RegField  reg_name=cfr_Params.BaseAddr + REG.Threshold  reg_rwmode=Read/Write  reg_msb=15  reg_lsb=0  reg_mode=Specify via dialog  reg_type=ufix(8)  reg_scale=2^-6  reg_init=cfr_Params.ClipVal  reg_desc=Clipping value  reg_modal=off  reg_desc0=0  reg_desc1=0  reg_desc2=0  reg_desc3=0  reg_desc4=0  reg_desc5=0  reg_desc6=0  reg_desc7=0  SampleTime=1  version=20090407
  Shift : DSPBAPrim/Shift  primtype=shift  nInputs=2  nOutputs=1  omode=Specify via dialog  otype=sfix(16)  scale=2^-15  rndmethod=Unbiased  factor=1  satmethod=Symmetric  shift_vec=[0 1 2 -1]  value=0  inPortNames=['a'; 'b';]  outPortNames=[' ']  dspbaimage=dspba_prim.jpg  text=fprintf('a >> b');  style=Optimised  visibilities=8  version=20090407
  Shift1 : DSPBAPrim/Shift  primtype=shift  nInputs=2  nOutputs=1  omode=Specify via dialog  otype=sfix(16)  scale=2^-15  rndmethod=Unbiased  factor=1  satmethod=Symmetric  shift_vec=[0 1 2 -1]  value=0  inPortNames=['a'; 'b';]  outPortNames=[' ']  dspbaimage=dspba_prim.jpg  text=fprintf('a >> b');  style=Optimised  visibilities=8  version=20090407
  Sub1 : DSPBAPrim/Sub  primtype=sub  nInputs=2  nOutputs=1  omode=Inherit via internal rule  otype=sfix(16)  scale=2^-15  rndmethod=Unbiased  factor=1  satmethod=Symmetric  shift_vec=[0 1 2 -1]  value=0  inPortNames=['+'; '-';]  outPortNames=[' ']  dspbaimage=dspba_prim.jpg  text=fprintf('-');  style=Optimised  visibilities=8  floatRounding=correct  advOptions=[]  version=20130115
  Subsystem : Subsystem  AncestorBlock=CORDIC_lib/Subsystem  mask{stages=8, angle_bits=16, angle_frac_bits=15, xy_bits=18, xy_frac_bits=14}
      mask prompts: angle_bits "Angle bits"; angle_frac_bits "Angle fractional bits"; xy_bits "XY bits"; xy_frac_bits "XY fractional bits"
      mask init:
      | sys = gcb;
      | 
      | % error trapping
      | if (angle_bits-angle_frac_bits)<3
      |     fprintf(['Warning (' sys ') not sufficient angle integer bits to represent full angle swing (-pi to pi)']);
      | end
      | 
      | if angle_bits < stages 
      |     fprintf(['Warning (' sys ') #angle bits < stages behaviour may be unexpected']);
      | end
      | 
      | if xy_bits < stages 
      |     fprintf(['Warning (' sys ') #xy bits < stages behaviour may be unexpected']);
      | end
      mask Display:
      | % calculate gain
      | gain = 1;
      | for i=0:stages
      |     gain = gain*(sqrt((1+2^(-2*i))));
      | end
      | color('w');image(imread('dspba_prim.jpg'));
      | fprintf('CORDIC\nRotate\n(pi to -pi)\ngain=%1.4f\niterations=%i',gain,stages+1);
      | port_label('input',1,'v_in');
      | port_label('input',2,'c_in');
      | port_label('input',3,'x_in');
      | port_label('input',4,'y_in');
      | port_label('input',5,'p_in');
      | port_label('output',1,'v_out');
      | port_label('output',2,'c_out');
      | port_label('output',3,'x_out');
      | port_label('output',4,'y_out');
      | port_label('output',5,'p_out');
  TermY{3..4,7..8} (4 alike) : Terminator
  qv : Outport
  qc : Outport  Port=2
  Out_c : Outport  Port=3
  r+i : Outport  Port=4
  wires:
  Add1/1 -> r+i/1
  Convert8/1 -> Mult1/2, Mult/2
  Mux/1 -> Convert8/1
  Real-Imag to Complex/1 -> Out_c/1
  c/1 -> qc/1
  v/1 -> qv/1
  d/1 -> Complex to Real-Iag/1
  Divide/1 -> Mux/2
  Const2/1 -> Mux/3
  Convert1/1 -> Real-Imag to Complex/2, Add1/2
  Convert/1 -> Add1/1, Real-Imag to Complex/1
  Convert6/1 -> Mult1/1
  Convert5/1 -> Mult/1
  Mult1/1 -> Convert1/1
  Mult/1 -> Convert/1
  RegField/1 -> Sub1/2
  BitExtract/1 -> Mux/1
  Sub1/1 -> BitExtract/1, Divide/1
  One2/1 -> Subsystem/5(pin)
  Subsystem/1(qv) -> TermY8/1
  Subsystem/2(qc) -> TermY7/1
  Subsystem/4(yout) -> TermY4/1
  Subsystem/5(pout) -> TermY3/1
  Convert10/1 -> Divide/2, Sub1/1
  Complex to Real-Iag/1 -> Convert5/1, Shift/1
  Complex to Real-Iag/2 -> Convert6/1, Shift1/1
  Shift/1 -> Subsystem/3(xin)
  Shift1/1 -> Subsystem/4(yin)
  One5/1 -> Shift/2, Shift1/2
  Subsystem/3(xout) -> Convert10/1
  One3/1 -> Subsystem/1(av)
  One4/1 -> Subsystem/2(ac)

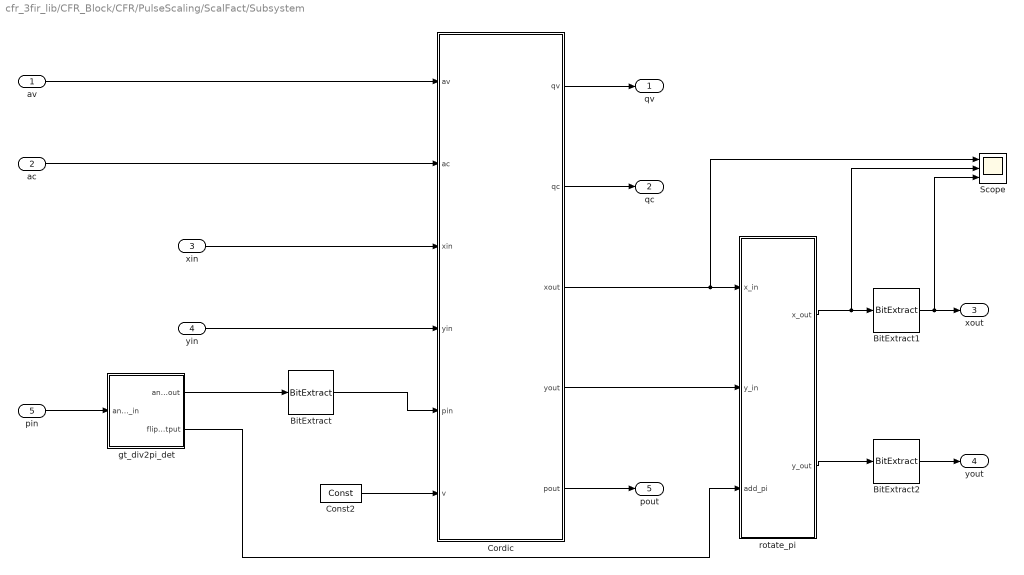
== system cfr_3fir_lib/CFR_Block/CFR/PulseScaling/ScalFact/Subsystem ==
  av : Inport
  ac : Inport  Port=2
  xin : Inport  Port=3
  yin : Inport  Port=4
  pin : Inport  Port=5
  BitExtract : DSPBAPrim/BitExtract  primtype=bitextract  nInputs=1  nOutputs=1  omode=Specify via dialog  otype=sfix(angle_bits-1)  scale=2^-angle_frac_bits  rndmethod=Unbiased  factor=1  satmethod=Symmetric  shift_vec=[0 1 2 -1]  value=0  inPortNames=[' '; ' ';]  outPortNames=[' ']  dspbaimage=dspba_prim.jpg  text=fprintf('..%d', value);  style=Optimised  visibilities=8 + 1024  version=20090407
  BitExtract1 : DSPBAPrim/BitExtract  primtype=bitextract  nInputs=1  nOutputs=1  omode=Specify via dialog  otype=sfix(xy_bits)  scale=2^-xy_frac_bits  rndmethod=Unbiased  factor=1  satmethod=Symmetric  shift_vec=[0 1 2 -1]  value=0  inPortNames=[' '; ' ';]  outPortNames=[' ']  dspbaimage=dspba_prim.jpg  text=fprintf('..%d', value);  style=Optimised  visibilities=8 + 1024  version=20090407
  BitExtract2 : DSPBAPrim/BitExtract  primtype=bitextract  nInputs=1  nOutputs=1  omode=Specify via dialog  otype=sfix(xy_bits)  scale=2^-xy_frac_bits  rndmethod=Unbiased  factor=1  satmethod=Symmetric  shift_vec=[0 1 2 -1]  value=0  inPortNames=[' '; ' ';]  outPortNames=[' ']  dspbaimage=dspba_prim.jpg  text=fprintf('..%d', value);  style=Optimised  visibilities=8 + 1024  version=20090407
  Const2 : DSPBAPrim/Const  primtype=const  nInputs=0  nOutputs=1  omode=Specify via dialog  otype=uint(1)  scale=2^0  rndmethod=Unbiased  factor=1  satmethod=Symmetric  shift_vec=[0 1 2 -1]  value=1  inPortNames=['+'; '+';]  outPortNames=[' ']  dspbaimage=dspba_prim.jpg  text=fprintf('%s', num2str(value));  style=Optimised  visibilities=8 + 1024  floatPrecision=float32_m23  version=20120820
  Cordic : Subsystem  AncestorBlock=CORDIC_lib/Cordic  mask(CORDIC range -pi/2 to pi/2){stages=stages, angle_bits=angle_bits-1, angle_frac_bits=angle_frac_bits, xy_bits=xy_bits, xy_frac_bits=xy_frac_bits}
      mask prompts: angle_bits "Angle bits"; angle_frac_bits "Angle fractional bits"; xy_bits "XY bits"; xy_frac_bits "XY fractional bits"
      mask help:
      | Primitive block implementation of CORDIC.
      | Range -pi/2 to pi/2
      |
      | See "Help" for information on parameter selection.
      mask init:
      | setup_cordic_block(stages, angle_bits, angle_frac_bits, xy_bits, xy_frac_bits);
      mask Help:
      | By default it is expected that stages = angle_bits = xy_bits also that
      | angle_frac_bits = angle_bits-2 (i.e. 2 integer angle bits)
      | 
      | It is assumed that stages <= angle_bits and stages <= xy_bits
      | 
      | Parameter description:
      | 
      | Stages (stages)
      | Number of CORDIC stages
      | Note counting starts at zero so "iterations = stages+1"
      | 
      | Angle bits (angle_bits)
      | Number of bits used to represent the angle, data format is "sfix"
      | 
      | Angle fractional bits (angle_frac_bits)
      | Number of angle bits which are fractional
      | Angle format will be "sfix[angle_bits]_[angle_frac_bits]"
      | 
      | XY bits (xy_bits)
      | Number of bits used to represent inputs x,y, data format is "sfix"
      | 
      | XY fractional bits (xy_frac_bits)
      | Number of x,y bits which are fractional
      | Format will be "sfix[xy_bits]_[xy_frac_bits]"
      | 
      | 
      | For more information on CORDIC see the following paper (from which this
      | implementation was created):
      | 
      | "A survey of CORDIC algorithms for FPGAs"
      | Ray Andraka, FPGA '98
      mask Display:
      | % calculate gain
      | gain = 1;
      | for i=0:stages
      |     gain = gain*(sqrt((1+2^(-2*i))));
      | end
      | color('w');image(imread('dspba_prim.jpg'));
      | fprintf('CORDIC\n(pi/2 to -pi/2)\ngain=%1.4f\niterations=%i',gain,stages+1);
      | 
      | port_label('input',1,'v_in');
      | port_label('input',2,'c_in');
      | port_label('input',3,'x_in');
      | port_label('input',4,'y_in');
      | port_label('input',5,'p_in');
      | port_label('input',6,'mode');
      | port_label('output',1,'v_out');
      | port_label('output',2,'c_out');
      | port_label('output',3,'x_out');
      | port_label('output',4,'y_out');
      | port_label('output',5,'p_out');
  Scope : Scope  NumInputPorts=3
  gt_div2pi_det : Subsystem  mask{angle_bits=angle_bits}
      mask prompts: angle_bits "Angle bits"
  rotate_pi : Subsystem
  qv : Outport
  qc : Outport  Port=2
  xout : Outport  Port=3
  yout : Outport  Port=4
  pout : Outport  Port=5
  wires:
  av/1 -> Cordic/1(av)
  ac/1 -> Cordic/2(ac)
  Cordic/1(qv) -> qv/1
  Cordic/2(qc) -> qc/1
  Cordic/3(xout) -> Scope/1, rotate_pi/1(x_in)
  Cordic/4(yout) -> rotate_pi/2(y_in)
  Cordic/5(pout) -> pout/1
  xin/1 -> Cordic/3(xin)
  yin/1 -> Cordic/4(yin)
  pin/1 -> gt_div2pi_det/1(angle_in)
  gt_div2pi_det/1(angle_out) -> BitExtract/1
  rotate_pi/1(x_out) -> Scope/2, BitExtract1/1
  rotate_pi/2(y_out) -> BitExtract2/1
  gt_div2pi_det/2(flip_output) -> rotate_pi/3(add_pi)
  Const2/1 -> Cordic/6(v)
  BitExtract/1 -> Cordic/5(pin)
  BitExtract1/1 -> Scope/3, xout/1
  BitExtract2/1 -> yout/1

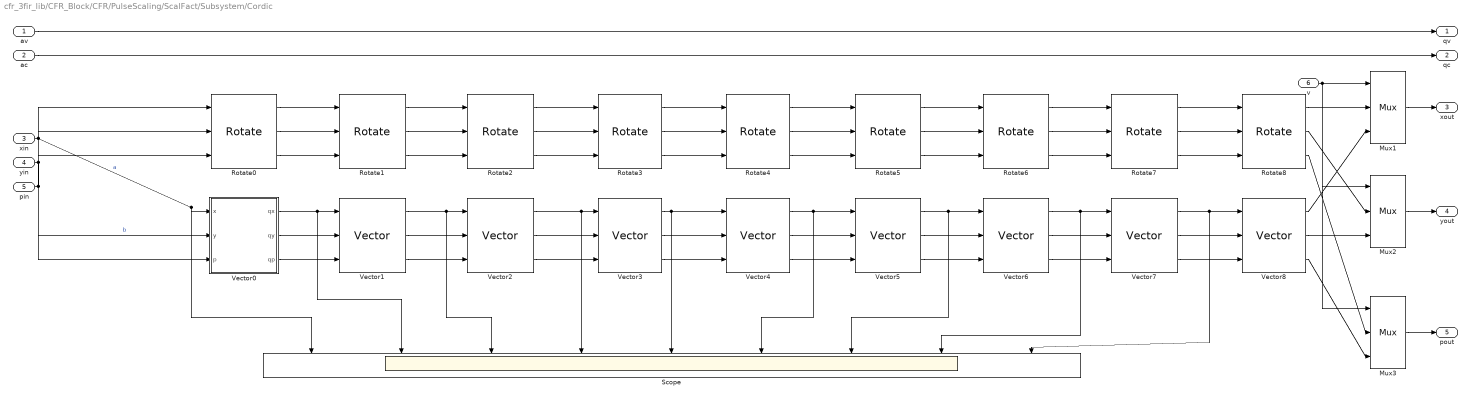
== system cfr_3fir_lib/CFR_Block/CFR/PulseScaling/ScalFact/Subsystem/Cordic ==
  av : Inport
  ac : Inport  Port=2
  xin : Inport  Port=3
  yin : Inport  Port=4
  pin : Inport  Port=5
  v : Inport  Port=6
  Mux1 : DSPBAPrim/Mux  primtype=mux  nInputs=evalAionMaskParam(gcb,'value',1)+1  nOutputs=1  omode=Inherit via internal rule  otype=sfix(16)  scale=2^-15  rndmethod=Unbiased  factor=1  satmethod=Symmetric  shift_vec=[0 1 2 -1]  value=2  inPortNames=['s'; 'd0'; 'd1'; 'd2'; 'd3'; 'd4'; 'd5'; 'd6'; 'd7'; 'd8'; 'd9';]  outPortNames=[' ']  dspbaimage=dspba_prim.jpg  text=fprintf('%s', primtype);  style=Optimised  visibilities=1032  version=20131025
  Mux2 : DSPBAPrim/Mux  primtype=mux  nInputs=evalAionMaskParam(gcb,'value',1)+1  nOutputs=1  omode=Inherit via internal rule  otype=sfix(16)  scale=2^-15  rndmethod=Unbiased  factor=1  satmethod=Symmetric  shift_vec=[0 1 2 -1]  value=2  inPortNames=['s'; 'd0'; 'd1'; 'd2'; 'd3'; 'd4'; 'd5'; 'd6'; 'd7'; 'd8'; 'd9';]  outPortNames=[' ']  dspbaimage=dspba_prim.jpg  text=fprintf('%s', primtype);  style=Optimised  visibilities=1032  version=20131025
  Mux3 : DSPBAPrim/Mux  primtype=mux  nInputs=evalAionMaskParam(gcb,'value',1)+1  nOutputs=1  omode=Inherit via internal rule  otype=sfix(16)  scale=2^-15  rndmethod=Unbiased  factor=1  satmethod=Symmetric  shift_vec=[0 1 2 -1]  value=2  inPortNames=['s'; 'd0'; 'd1'; 'd2'; 'd3'; 'd4'; 'd5'; 'd6'; 'd7'; 'd8'; 'd9';]  outPortNames=[' ']  dspbaimage=dspba_prim.jpg  text=fprintf('%s', primtype);  style=Optimised  visibilities=1032  version=20131025
  Rotate0 : CORDIC_lib/Rotate  stage=0  angle_bits=15  angle_frac_bits=15  xy_bits=18  xy_frac_bits=14
  Rotate1 : CORDIC_lib/Rotate  stage=1  angle_bits=15  angle_frac_bits=15  xy_bits=18  xy_frac_bits=14
  Rotate2 : CORDIC_lib/Rotate  stage=2  angle_bits=15  angle_frac_bits=15  xy_bits=18  xy_frac_bits=14
  Rotate3 : CORDIC_lib/Rotate  stage=3  angle_bits=15  angle_frac_bits=15  xy_bits=18  xy_frac_bits=14
  Rotate4 : CORDIC_lib/Rotate  stage=4  angle_bits=15  angle_frac_bits=15  xy_bits=18  xy_frac_bits=14
  Rotate5 : CORDIC_lib/Rotate  stage=5  angle_bits=15  angle_frac_bits=15  xy_bits=18  xy_frac_bits=14
  Rotate6 : CORDIC_lib/Rotate  stage=6  angle_bits=15  angle_frac_bits=15  xy_bits=18  xy_frac_bits=14
  Rotate7 : CORDIC_lib/Rotate  stage=7  angle_bits=15  angle_frac_bits=15  xy_bits=18  xy_frac_bits=14
  Rotate8 : CORDIC_lib/Rotate  stage=8  angle_bits=15  angle_frac_bits=15  xy_bits=18  xy_frac_bits=14
  Scope : Scope  NumInputPorts=9
  Vector0 : Subsystem  AncestorBlock=CORDIC_lib/Vector  mask{stage=0, angle_bits=15, angle_frac_bits=15, xy_bits=18, xy_frac_bits=14}
      mask prompts: angle_bits "Angle bits"; angle_frac_bits "Angle fractional bits"; xy_bits "XY bits"; xy_frac_bits "XY fractional bits"
  Vector1 : CORDIC_lib/Vector  stage=1  angle_bits=15  angle_frac_bits=15  xy_bits=18  xy_frac_bits=14
  Vector2 : CORDIC_lib/Vector  stage=2  angle_bits=15  angle_frac_bits=15  xy_bits=18  xy_frac_bits=14
  Vector3 : CORDIC_lib/Vector  stage=3  angle_bits=15  angle_frac_bits=15  xy_bits=18  xy_frac_bits=14
  Vector4 : CORDIC_lib/Vector  stage=4  angle_bits=15  angle_frac_bits=15  xy_bits=18  xy_frac_bits=14
  Vector5 : CORDIC_lib/Vector  stage=5  angle_bits=15  angle_frac_bits=15  xy_bits=18  xy_frac_bits=14
  Vector6 : CORDIC_lib/Vector  stage=6  angle_bits=15  angle_frac_bits=15  xy_bits=18  xy_frac_bits=14
  Vector7 : CORDIC_lib/Vector  stage=7  angle_bits=15  angle_frac_bits=15  xy_bits=18  xy_frac_bits=14
  Vector8 : CORDIC_lib/Vector  stage=8  angle_bits=15  angle_frac_bits=15  xy_bits=18  xy_frac_bits=14
  qv : Outport
  qc : Outport  Port=2
  xout : Outport  Port=3
  yout : Outport  Port=4
  pout : Outport  Port=5
  wires:
  av/1 -> qv/1
  ac/1 -> qc/1
  xin/1 -> Rotate0/1, Scope/1, Vector0/1(x)  "a"
  yin/1 -> Rotate0/2, Vector0/2(y)  "b"
  pin/1 -> Rotate0/3, Vector0/3(p)
  Rotate0/1 -> Rotate1/1
  Vector0/1(qx) -> Scope/2, Vector1/1
  Rotate0/2 -> Rotate1/2
  Vector0/2(qy) -> Vector1/2
  Rotate0/3 -> Rotate1/3
  Vector0/3(qp) -> Vector1/3
  Rotate1/1 -> Rotate2/1
  Vector1/1 -> Scope/3, Vector2/1
  Rotate1/2 -> Rotate2/2
  Vector1/2 -> Vector2/2
  Rotate1/3 -> Rotate2/3
  Vector1/3 -> Vector2/3
  Rotate2/1 -> Rotate3/1
  Vector2/1 -> Scope/4, Vector3/1
  Rotate2/2 -> Rotate3/2
  Vector2/2 -> Vector3/2
  Rotate2/3 -> Rotate3/3
  Vector2/3 -> Vector3/3
  Rotate3/1 -> Rotate4/1
  Vector3/1 -> Vector4/1, Scope/5
  Rotate3/2 -> Rotate4/2
  Vector3/2 -> Vector4/2
  Rotate3/3 -> Rotate4/3
  Vector3/3 -> Vector4/3
  Rotate4/1 -> Rotate5/1
  Vector4/1 -> Scope/6, Vector5/1
  Rotate4/2 -> Rotate5/2
  Vector4/2 -> Vector5/2
  Rotate4/3 -> Rotate5/3
  Vector4/3 -> Vector5/3
  Rotate5/1 -> Rotate6/1
  Vector5/1 -> Scope/7, Vector6/1
  Rotate5/2 -> Rotate6/2
  Vector5/2 -> Vector6/2
  Rotate5/3 -> Rotate6/3
  Vector5/3 -> Vector6/3
  Rotate6/1 -> Rotate7/1
  Vector6/1 -> Scope/8, Vector7/1
  Rotate6/2 -> Rotate7/2
  Vector6/2 -> Vector7/2
  Rotate6/3 -> Rotate7/3
  Vector6/3 -> Vector7/3
  Rotate7/1 -> Rotate8/1
  Vector7/1 -> Scope/9, Vector8/1
  Rotate7/2 -> Rotate8/2
  Vector7/2 -> Vector8/2
  Rotate7/3 -> Rotate8/3
  Vector7/3 -> Vector8/3
  v/1 -> Mux1/1, Mux2/1, Mux3/1
  Rotate8/1 -> Mux1/2
  Vector8/1 -> Mux1/3
  Rotate8/2 -> Mux2/2
  Vector8/2 -> Mux2/3
  Rotate8/3 -> Mux3/2
  Vector8/3 -> Mux3/3
  Mux1/1 -> xout/1
  Mux2/1 -> yout/1
  Mux3/1 -> pout/1
